simulink model "embeddedM_example"  (R2018a)
settings: Solver=FixedStepDiscrete  StartTime=0.0  StopTime=10.0  RelTol=1e-3
settings Model: Creator=wolfgang  LastModifiedBy=oskwij-4

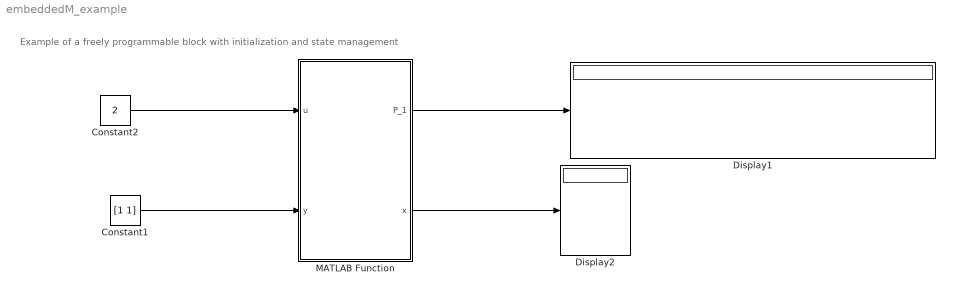
== system embeddedM_example ==
  note: Example of a freely programmable block with initialization and state management
  Constant1 : Constant  Value=[1 1]
  Constant2 : Constant  Value=2
  Display1 : Display
  Display2 : Display
  MATLAB Function : MATLAB Function  TreatAsAtomicUnit=on
  wires:
  MATLAB Function/2(x) -> Display2/1
  MATLAB Function/1(P_1) -> Display1/1
  Constant2/1 -> MATLAB Function/1(u)
  Constant1/1 -> MATLAB Function/2(y)

== matlab function embeddedM_example/MATLAB Function ==
  data: u input; y input; P_1 output; x output
function [P_1,x] = fcn(u,y)
persistent P_0;
 if isempty(P_0)
        P_0  = [8 8;8 8];
 end
 persistent A_k;
 if isempty(A_k)
        A_k  = [0.991845657443151 0;0.008121005167024 0.991845657417614];
 end
  persistent B_k;
 if isempty(B_k)
        B_k  = [0.001912051102508;7.817036422671138e-06];
 end
  persistent C_k;
 if isempty(C_k)
        C_k  = [0 1];
 end
 persistent N_k;
 if isempty(N_k)
        N_k  = [0 1];
 end
 persistent Q_k;
 if isempty(Q_k)
        Q_k  = [1 0;0 1];
 end
 persistent R_k;
 if isempty(R_k)
        R_k  = [1 0;0 1];
 end
persistent x_0;
 if isempty(x_0)
     x_0 = [0 ; 0];
 end
persistent k_0;
 if isempty(k_0)
    k_0 = 0;
 end
 
x_hat = A_k*x_0+B_k*u;
P = A_k*P_0*A_k'+N_k*Q_k*N_k';

K = P*(C_k')\(((C_k*P)*C_k')+R_k);
y_k = y-C_k*x_hat;
x = x_hat+K*y_k;
P_1 = P-K*C_k*P;
